simulink model "untitled1"  (R2015a)
settings: Solver=ode45  StartTime=0.0  StopTime=10.0  RelTol=1e-3
libraries: dsparch4 x1
settings Model: Creator=TaD  LastModifiedBy=TaD

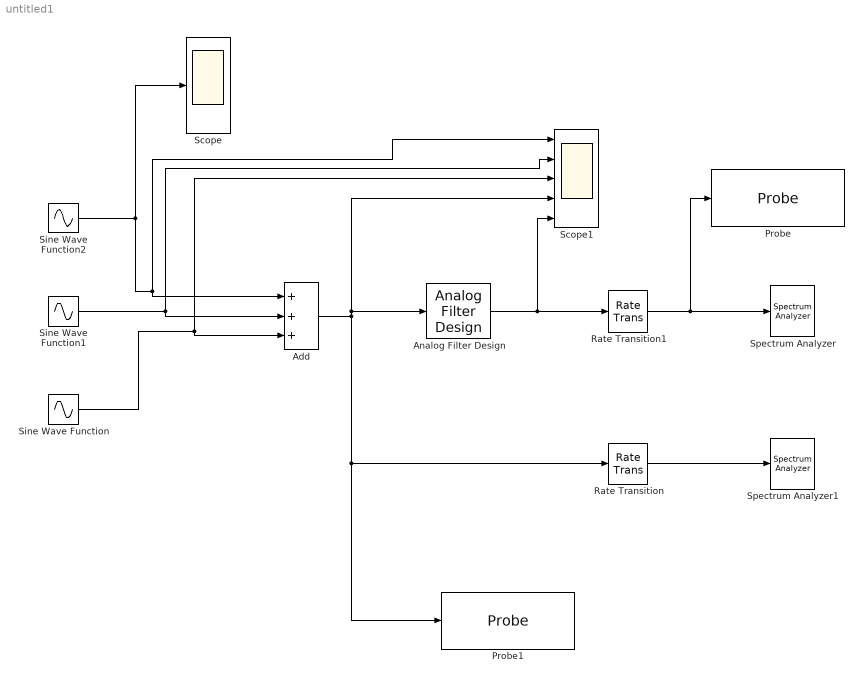
== system untitled1 ==
  Add : Sum  Inputs=+++
  Analog Filter Design : dsparch4/Analog Filter Design  method=Butterworth  filttype=Lowpass  N=9  Wlo=5000*pi  Whi=80  Rp=2  Rs=40
  Probe : Probe  ProbeSignalDimensions=on  ProbeFramedSignal=on
  Probe1 : Probe  ProbeSignalDimensions=on  ProbeFramedSignal=on
  Rate Transition : RateTransition  Deterministic=off  OutPortSampleTime=1/262144
  Rate Transition1 : RateTransition  Deterministic=off  OutPortSampleTime=1/262144
  Scope : Scope
  Scope1 : Scope  NumInputPorts=5
      settings: YMin=-5~-5~-5~-5~-5  YMax=5~5~5~5~5
  Sine Wave Function : Sin  Amplitude=2  Frequency=1000*pi  SampleTime=1e-5
  Sine Wave Function1 : Sin  Amplitude=2  Frequency=1000*pi  SampleTime=1e-5
  Sine Wave Function2 : Sin  Amplitude=2  Frequency=1000*pi  SampleTime=1e-5
  Spectrum Analyzer : SpectrumAnalyzer
  Spectrum Analyzer1 : SpectrumAnalyzer
  wires:
  Sine Wave Function2/1 -> Scope/1, Scope1/1, Add/1
  Sine Wave Function1/1 -> Scope1/2, Add/2
  Sine Wave Function/1 -> Scope1/3, Add/3
  Add/1 -> Scope1/4, Analog Filter Design/1, Rate Transition/1, Probe1/1
  Analog Filter Design/1 -> Scope1/5, Rate Transition1/1
  Rate Transition/1 -> Spectrum Analyzer1/1
  Rate Transition1/1 -> Probe/1, Spectrum Analyzer/1
